simulink model "Ser2G"  (R2012b)
settings: Solver=ode45  StartTime=0.0  StopTime=10.0  RelTol=1e-3
undefined symbols (not defined in the file or in its folder): Ser2
settings Model: Creator=Daniel  LastModifiedBy=Daniel

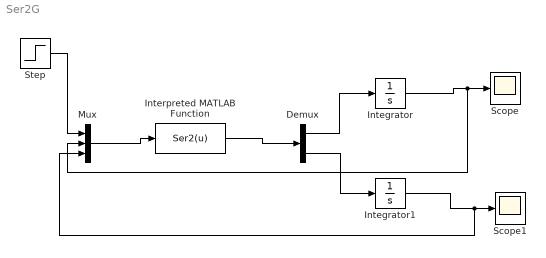
== system Ser2G ==
  Demux : Demux  Outputs=2
  Integrator : Integrator
  Integrator1 : Integrator
  Interpreted MATLAB Function : MATLABFcn  MATLABFcn=Ser2(u)  OutputDimensions=2
  Mux : Mux  Inputs=3
  Scope : Scope
  Scope1 : Scope
  Step : Step  After=3  SampleTime=0
  wires:
  Step/1 -> Mux/1
  Mux/1 -> Interpreted MATLAB Function/1
  Interpreted MATLAB Function/1 -> Demux/1
  Demux/1 -> Integrator/1
  Demux/2 -> Integrator1/1
  Integrator/1 -> Mux/2, Scope/1
  Integrator1/1 -> Mux/3, Scope1/1
